simulink model "Swerve_Module"  (R2023a)
settings: Solver=VariableStepAuto  StartTime=0.0  StopTime=10.0  RelTol=1e-3
model workspace (MAT data in the model file):
  Turn_Offset = 2
libraries: slpidlib x2, Rotation2D x2
settings Model: Creator=FIRSTMentor  LastModifiedBy=FIRSTMentor

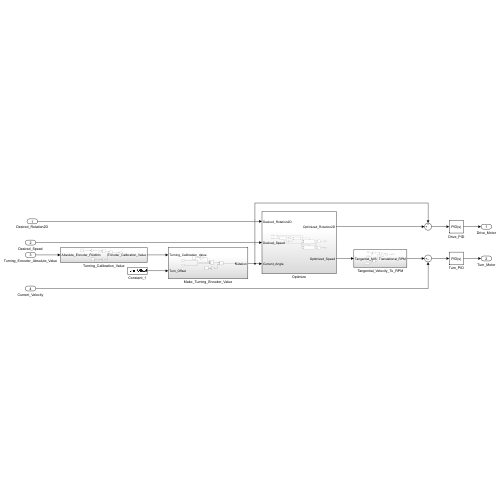
[thumbnail: Simulink's stored preview of the top-level diagram]
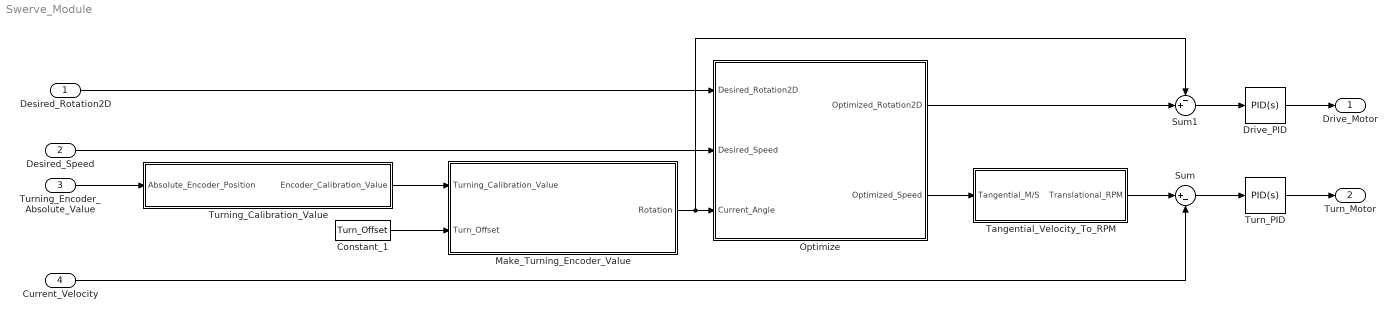
== system Swerve_Module ==
  Desired_Rotation2D : Inport  OutDataTypeStr=double  Unit=rad
  Desired_Speed : Inport  Port=2  OutDataTypeStr=double  Unit=m/s
  Turning_Encoder_Absolute_Value : Inport  Port=3  OutDataTypeStr=double  Unit=rad
  Current_Velocity : Inport  Port=4  OutDataTypeStr=double  Unit=m/s
  Constant_1 : Constant  Value=Turn_Offset
  Drive_PID : slpidlib/PID Controller  Controller=PID  Form=Parallel  TimeDomain=Continuous-time  UseExternalTs=off  SampleTime=-1  IntegratorMethod=Forward Euler  FilterMethod=Forward Euler  ControllerParametersSource=internal  P=1  I=1  UseKiTs=off  D=0  N=100  UseFilter=on  TunerSelectOption=Transfer Function Based (PID Tuner App)  InitialConditionSource=internal  InitialConditionForIntegrator=0  InitialConditionForFilter=0  DifferentiatorICPrevScaledInput=0  ExternalReset=none  TrackingMode=off  Kt=1  LimitOutput=off  SatLimitsSource=internal  UpperSaturationLimit=inf  LowerSaturationLimit=-inf  LinearizeAsGain=on  AntiWindupMode=none  Kb=1  LimitIntegrator=off  UpperIntegratorSaturationLimit=inf  LowerIntegratorSaturationLimit=-inf  POutMin=[]  POutMax=[]  IOutMin=[]  IOutMax=[]  DOutMin=[]  DOutMax=[]  NOutMin=[]  NOutMax=[]  SumOutMin=[]  SumOutMax=[]  SaturationOutMin=[]  SaturationOutMax=[]  PParamMin=[]  PParamMax=[]  IParamMin=[]  IParamMax=[]  DParamMin=[]  DParamMax=[]  NParamMin=[]  NParamMax=[]  KbParamMin=[]  KbParamMax=[]  KtParamMin=[]  KtParamMax=[]  KbOutMin=[]  KbOutMax=[]  KtOutMin=[]  KtOutMax=[]  IntegratorOutMin=[]  IntegratorOutMax=[]  FilterOutMin=[]  FilterOutMax=[]  SumI1OutMin=[]  SumI1OutMax=[]  SumI2OutMin=[]  SumI2OutMax=[]  SumI3OutMin=[]  SumI3OutMax=[]  SumI4OutMin=[]  SumI4OutMax=[]  SumDOutMin=[]  SumDOutMax=[]  DifferentiatorOutMin=[]  DifferentiatorOutMax=[]  FilterDiffOutCoefMin=[]  FilterDiffOutCoefMax=[]  ReciprocalOutMin=[]  ReciprocalOutMax=[]  SumDenOutMin=[]  SumDenOutMax=[]  SumNumOutMin=[]  SumNumOutMax=[]  DivideOutMin=[]  DivideOutMax=[]  UdiffTsProdOutMin=[]  UdiffTsProdOutMax=[]  NTsProdOutMin=[]  NTsProdOutMax=[]  UintegralTsProdOutMin=[]  UintegralTsProdOutMax=[]  UngainTsProdOutMin=[]  UngainTsProdOutMax=[]  ClampingZeroOutDataTypeStr=Inherit: Inherit via back propagation  ClampingZeroOutMin=[]  ClampingZeroOutMax=[]  FilterDenConstantOutDataTypeStr=Inherit: Inherit via back propagation  FilterDenConstantOutMin=[]  FilterDenConstantOutMax=[]  PCopyOutDataTypeStr=Inherit: Inherit via back propagation  PCopyOutMin=[]  PCopyOutMax=[]  NCopyOutDataTypeStr=Inherit: Inherit via back propagation  NCopyOutMin=[]  NCopyOutMax=[]  IntegratorContinuousStateAttributes=''  IntegratorStateMustResolveToSignalObject=off  IntegratorRTWStateStorageClass=Auto  FilterContinuousStateAttributes=''  FilterStateMustResolveToSignalObject=off  FilterRTWStateStorageClass=Auto  ParallelPVariant=InternalParameters  IdealPVariant=Disabled  IVariant=InternalParameters  DVariant=InternalParameters  IntegratorVariant=Continuous  SatVariant=Disabled  AWVariant=Passthrough  PCopyVariant=Disabled  TRVariant=Disabled  FdbkBlocksVariant=Forward  IdealPFdbkVariant=Disabled  SatFdbkVariant=Disabled  DerivativeFilterVariant=ContFilter  NVariant=InternalParameters  NCopyVariant=Disabled  FilterICVariant=InternalICsFilter  IntegratorICVariant=InternalICs  ExternalResetVariant=Disabled  TRSumVariant=Passthrough  SumFdbkVariant=Disabled  SumVariant=Sum_PID  TsampFilterVariant=InternalTs  TsampNgainVariant=Passthrough  TsampIntegralVariant=Disabled_SignalSpec  ExternalSaturationOutDataTypeStr=Inherit: Same as second input
  Make_Turning_Encoder_Value : Subsystem
  Optimize : Subsystem
  Sum : Sum  Inputs=|+-
  Sum1 : Sum  Inputs=-+|
  Tangential_Velocity_To_RPM : Subsystem
  Turn_PID : slpidlib/PID Controller  Controller=PID  Form=Parallel  TimeDomain=Continuous-time  UseExternalTs=off  SampleTime=-1  IntegratorMethod=Forward Euler  FilterMethod=Forward Euler  ControllerParametersSource=internal  P=1  I=1  UseKiTs=off  D=0  N=100  UseFilter=on  TunerSelectOption=Transfer Function Based (PID Tuner App)  InitialConditionSource=internal  InitialConditionForIntegrator=0  InitialConditionForFilter=0  DifferentiatorICPrevScaledInput=0  ExternalReset=none  TrackingMode=off  Kt=1  LimitOutput=off  SatLimitsSource=internal  UpperSaturationLimit=inf  LowerSaturationLimit=-inf  LinearizeAsGain=on  AntiWindupMode=none  Kb=1  LimitIntegrator=off  UpperIntegratorSaturationLimit=inf  LowerIntegratorSaturationLimit=-inf  POutMin=[]  POutMax=[]  IOutMin=[]  IOutMax=[]  DOutMin=[]  DOutMax=[]  NOutMin=[]  NOutMax=[]  SumOutMin=[]  SumOutMax=[]  SaturationOutMin=[]  SaturationOutMax=[]  PParamMin=[]  PParamMax=[]  IParamMin=[]  IParamMax=[]  DParamMin=[]  DParamMax=[]  NParamMin=[]  NParamMax=[]  KbParamMin=[]  KbParamMax=[]  KtParamMin=[]  KtParamMax=[]  KbOutMin=[]  KbOutMax=[]  KtOutMin=[]  KtOutMax=[]  IntegratorOutMin=[]  IntegratorOutMax=[]  FilterOutMin=[]  FilterOutMax=[]  SumI1OutMin=[]  SumI1OutMax=[]  SumI2OutMin=[]  SumI2OutMax=[]  SumI3OutMin=[]  SumI3OutMax=[]  SumI4OutMin=[]  SumI4OutMax=[]  SumDOutMin=[]  SumDOutMax=[]  DifferentiatorOutMin=[]  DifferentiatorOutMax=[]  FilterDiffOutCoefMin=[]  FilterDiffOutCoefMax=[]  ReciprocalOutMin=[]  ReciprocalOutMax=[]  SumDenOutMin=[]  SumDenOutMax=[]  SumNumOutMin=[]  SumNumOutMax=[]  DivideOutMin=[]  DivideOutMax=[]  UdiffTsProdOutMin=[]  UdiffTsProdOutMax=[]  NTsProdOutMin=[]  NTsProdOutMax=[]  UintegralTsProdOutMin=[]  UintegralTsProdOutMax=[]  UngainTsProdOutMin=[]  UngainTsProdOutMax=[]  ClampingZeroOutDataTypeStr=Inherit: Inherit via back propagation  ClampingZeroOutMin=[]  ClampingZeroOutMax=[]  FilterDenConstantOutDataTypeStr=Inherit: Inherit via back propagation  FilterDenConstantOutMin=[]  FilterDenConstantOutMax=[]  PCopyOutDataTypeStr=Inherit: Inherit via back propagation  PCopyOutMin=[]  PCopyOutMax=[]  NCopyOutDataTypeStr=Inherit: Inherit via back propagation  NCopyOutMin=[]  NCopyOutMax=[]  IntegratorContinuousStateAttributes=''  IntegratorStateMustResolveToSignalObject=off  IntegratorRTWStateStorageClass=Auto  FilterContinuousStateAttributes=''  FilterStateMustResolveToSignalObject=off  FilterRTWStateStorageClass=Auto  ParallelPVariant=InternalParameters  IdealPVariant=Disabled  IVariant=InternalParameters  DVariant=InternalParameters  IntegratorVariant=Continuous  SatVariant=Disabled  AWVariant=Passthrough  PCopyVariant=Disabled  TRVariant=Disabled  FdbkBlocksVariant=Forward  IdealPFdbkVariant=Disabled  SatFdbkVariant=Disabled  DerivativeFilterVariant=ContFilter  NVariant=InternalParameters  NCopyVariant=Disabled  FilterICVariant=InternalICsFilter  IntegratorICVariant=InternalICs  ExternalResetVariant=Disabled  TRSumVariant=Passthrough  SumFdbkVariant=Disabled  SumVariant=Sum_PID  TsampFilterVariant=InternalTs  TsampNgainVariant=Passthrough  TsampIntegralVariant=Disabled_SignalSpec  ExternalSaturationOutDataTypeStr=Inherit: Same as second input
  Turning_Calibration_Value : Subsystem
  Drive_Motor : Outport  OutDataTypeStr=double  Unit=1
  Turn_Motor : Outport  Port=2  OutDataTypeStr=double  Unit=1
  wires:
  Desired_Rotation2D/1 -> Optimize/1(Desired_Rotation2D)
  Turning_Calibration_Value/1(Encoder_Calibration_Value) -> Make_Turning_Encoder_Value/1(Turning_Calibration_Value)
  Make_Turning_Encoder_Value/1(Rotation) -> Sum1/1, Optimize/3(Current_Angle)
  Desired_Speed/1 -> Optimize/2(Desired_Speed)
  Sum1/1 -> Drive_PID/1
  Optimize/1(Optimized_Rotation2D) -> Sum1/2
  Current_Velocity/1 -> Sum/2
  Turning_Encoder_Absolute_Value/1 -> Turning_Calibration_Value/1(Absolute_Encoder_Position)
  Constant_1/1 -> Make_Turning_Encoder_Value/2(Turn_Offset)
  Drive_PID/1 -> Drive_Motor/1
  Turn_PID/1 -> Turn_Motor/1
  Optimize/2(Optimized_Speed) -> Tangential_Velocity_To_RPM/1(Tangential_M/S)
  Tangential_Velocity_To_RPM/1(Translational_RPM) -> Sum/1
  Sum/1 -> Turn_PID/1

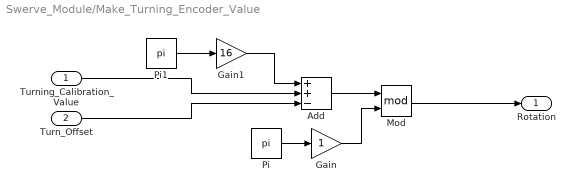
== system Swerve_Module/Make_Turning_Encoder_Value ==
  Turning_Calibration_Value : Inport  OutDataTypeStr=double  Unit=1
  Turn_Offset : Inport  Port=2  OutDataTypeStr=double  Unit=rad
  Add : Sum  Inputs=++-
  Gain : Gain
  Gain1 : Gain  Gain=16
  Mod : Math  Operator=mod
  Pi : Constant  Value=pi  OutDataTypeStr=Inherit: Inherit via back propagation
  Pi1 : Constant  Value=pi  OutDataTypeStr=Inherit: Inherit via back propagation
  Rotation : Outport  OutDataTypeStr=double  Unit=rad
  wires:
  Pi/1 -> Gain/1
  Gain/1 -> Mod/2
  Mod/1 -> Rotation/1
  Pi1/1 -> Gain1/1
  Gain1/1 -> Add/1
  Add/1 -> Mod/1
  Turning_Calibration_Value/1 -> Add/2
  Turn_Offset/1 -> Add/3

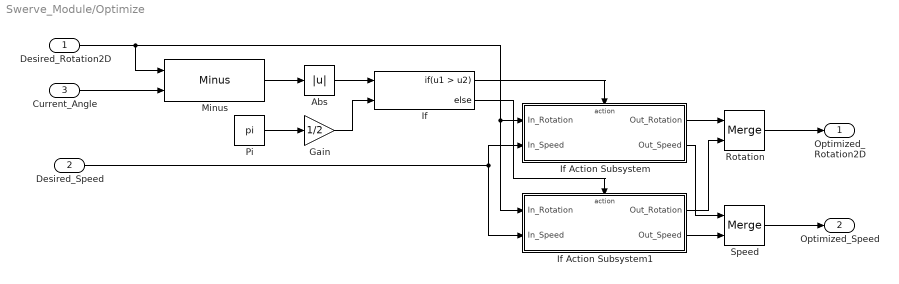
== system Swerve_Module/Optimize ==
  Desired_Rotation2D : Inport  OutDataTypeStr=double  Unit=rad
  Desired_Speed : Inport  Port=2  OutDataTypeStr=double  Unit=m/s
  Current_Angle : Inport  Port=3  OutDataTypeStr=double  Unit=rad
  Abs : Abs  SaturateOnIntegerOverflow=off
  Gain : Gain  Gain=1/2
  If : If  NumInputs=2  IfExpression=u1 > u2
  If Action Subsystem : Subsystem  TreatAsAtomicUnit=on
  If Action Subsystem1 : Subsystem  TreatAsAtomicUnit=on
  Minus : Rotation2D/Minus  SystemSampleTime=-1  VariantActivationTime=update diagram  Latency=0  AutoFrameSizeCalculation=off
  Pi : Constant  Value=pi  OutDataTypeStr=Inherit: Inherit via back propagation
  Rotation : Merge
  Speed : Merge
  Optimized_Rotation2D : Outport  OutDataTypeStr=double  Unit=rad
  Optimized_Speed : Outport  Port=2  OutDataTypeStr=double  Unit=m/s
  wires:
  Pi/1 -> Gain/1
  Desired_Rotation2D/1 -> If Action Subsystem/1(In_Rotation), If Action Subsystem1/1(In_Rotation), Minus/1
  Current_Angle/1 -> Minus/2
  Minus/1 -> Abs/1
  If Action Subsystem1/2(Out_Speed) -> Speed/2
  Gain/1 -> If/2
  Abs/1 -> If/1
  If/1 -> If Action Subsystem/Action
  If/2 -> If Action Subsystem1/Action
  If Action Subsystem1/1(Out_Rotation) -> Rotation/2
  Desired_Speed/1 -> If Action Subsystem/2(In_Speed), If Action Subsystem1/2(In_Speed)
  If Action Subsystem/1(Out_Rotation) -> Rotation/1
  If Action Subsystem/2(Out_Speed) -> Speed/1
  Rotation/1 -> Optimized_Rotation2D/1
  Speed/1 -> Optimized_Speed/1

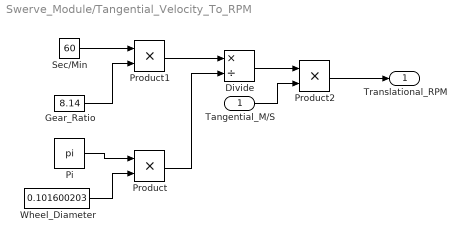
== system Swerve_Module/Tangential_Velocity_To_RPM ==
  Tangential_M/S : Inport
  Divide : Product  Inputs=*/
  Gear_Ratio : Constant  Value=8.14
  Pi : Constant  Value=pi  OutDataTypeStr=Inherit: Inherit via back propagation
  Product : Product
  Product1 : Product
  Product2 : Product
  Sec/Min : Constant  Value=60
  Wheel_Diameter : Constant  Value=0.101600203
  Translational_RPM : Outport
  wires:
  Product/1 -> Divide/2
  Pi/1 -> Product/1
  Product1/1 -> Divide/1
  Sec/Min/1 -> Product1/1
  Gear_Ratio/1 -> Product1/2
  Divide/1 -> Product2/1
  Product2/1 -> Translational_RPM/1
  Tangential_M/S/1 -> Product2/2
  Wheel_Diameter/1 -> Product/2

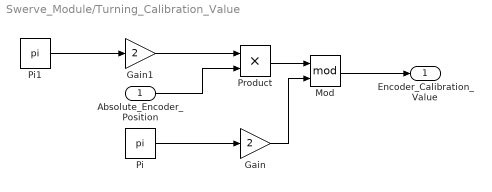
== system Swerve_Module/Turning_Calibration_Value ==
  Absolute_Encoder_Position : Inport  OutDataTypeStr=double  Unit=rad
  Gain : Gain  Gain=2
  Gain1 : Gain  Gain=2
  Mod : Math  Operator=mod
  Pi : Constant  Value=pi  OutDataTypeStr=Inherit: Inherit via back propagation
  Pi1 : Constant  Value=pi  OutDataTypeStr=Inherit: Inherit via back propagation
  Product : Product
  Encoder_Calibration_Value : Outport  OutDataTypeStr=double  Unit=1
  wires:
  Mod/1 -> Encoder_Calibration_Value/1
  Gain/1 -> Mod/2
  Product/1 -> Mod/1
  Pi1/1 -> Gain1/1
  Pi/1 -> Gain/1
  Absolute_Encoder_Position/1 -> Product/2
  Gain1/1 -> Product/1

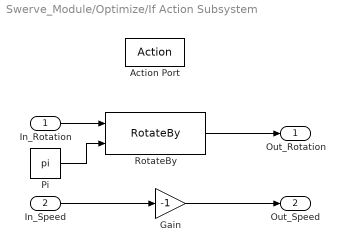
== system Swerve_Module/Optimize/If Action Subsystem ==
  In_Rotation : Inport  OutDataTypeStr=double  Unit=rad
  In_Speed : Inport  Port=2  OutDataTypeStr=double  Unit=m/s
  Action Port : ActionPort  ActionPortLabel=if(u1 > u2)
  Gain : Gain  Gain=-1
  Pi : Constant  Value=pi  OutDataTypeStr=Inherit: Inherit via back propagation
  RotateBy : Rotation2D/RotateBy  SystemSampleTime=-1  VariantActivationTime=update diagram  Latency=0  AutoFrameSizeCalculation=off
  Out_Rotation : Outport  OutDataTypeStr=double  Unit=rad
  Out_Speed : Outport  Port=2  OutDataTypeStr=double  Unit=m/s
  wires:
  In_Speed/1 -> Gain/1
  Gain/1 -> Out_Speed/1
  In_Rotation/1 -> RotateBy/1
  RotateBy/1 -> Out_Rotation/1
  Pi/1 -> RotateBy/2

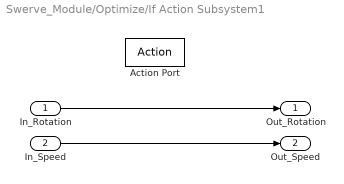
== system Swerve_Module/Optimize/If Action Subsystem1 ==
  In_Rotation : Inport  OutDataTypeStr=double  Unit=rad
  In_Speed : Inport  Port=2  OutDataTypeStr=double  Unit=m/s
  Action Port : ActionPort  ActionPortLabel=else
  Out_Rotation : Outport  OutDataTypeStr=double  Unit=rad
  Out_Speed : Outport  Port=2  OutDataTypeStr=double  Unit=m/s
  wires:
  In_Rotation/1 -> Out_Rotation/1
  In_Speed/1 -> Out_Speed/1
